simulink model "Week6"  (R2020b)
settings: Solver=VariableStepAuto  StartTime=0.0  StopTime=5  MaxStep=1e-4  RelTol=1e-3
undefined symbols (not defined in the file or in its folder): Capacitor, Run, Start
libraries: powerlib x9
settings Model: Creator=emman  LastModifiedBy=emman

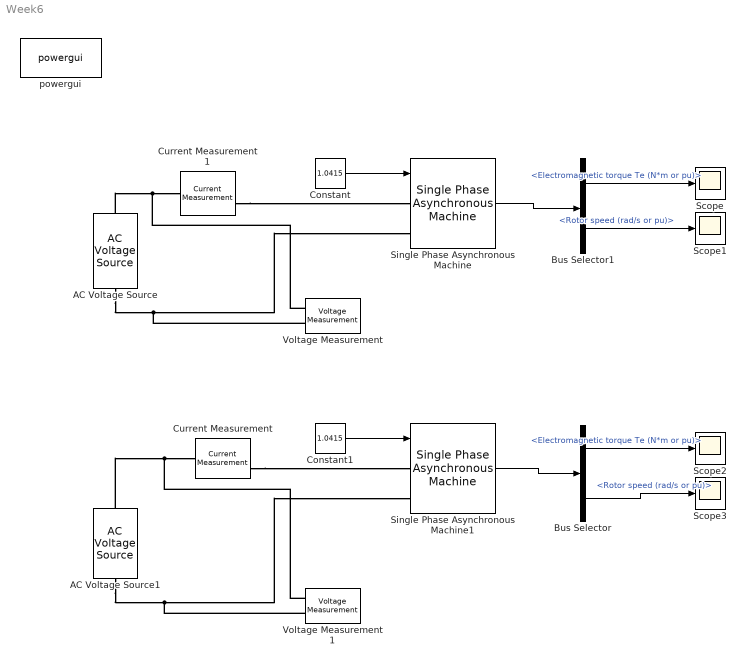
== system Week6 ==
  AC Voltage Source : powerlib/Electrical Sources/AC Voltage Source  Amplitude=110*sqrt(2)  Phase=90  Frequency=60  SampleTime=0  Measurements=None  BusType=swing  Pref=10e3  Qref=0  Qmin=-inf  Qmax=+inf
  AC Voltage Source1 : powerlib/Electrical Sources/AC Voltage Source  Amplitude=110*sqrt(2)  Phase=90  Frequency=60  SampleTime=0  Measurements=None  BusType=swing  Pref=10e3  Qref=0  Qmin=-inf  Qmax=+inf
  Bus Selector : BusSelector  OutputSignals=Mechanical.Electromagnetic torque Te (N*m or pu),Mechanical.Rotor speed (rad/s or pu)
  Bus Selector1 : BusSelector  OutputSignals=Mechanical.Electromagnetic torque Te (N*m or pu),Mechanical.Rotor speed (rad/s or pu)
  Constant : Constant  Value=1.0415
  Constant1 : Constant  Value=1.0415
  Current Measurement : powerlib/Measurements/Current Measurement  PhasorSimulation=off  OutputType=Complex  PSBequivalent=0
  Current Measurement1 : powerlib/Measurements/Current Measurement  PhasorSimulation=off  OutputType=Complex  PSBequivalent=0
  Scope{,1..3} (4 alike) : Scope
  Single Phase Asynchronous Machine : powerlib/Machines/Single Phase Asynchronous Machine  MechanicalLoad=Torque Tm  UNITS=SI  MachineType=Capacitor-Start  MeasurementBus=off  NominalParameters="[0.25*746  110  60]"  MainWindingStator="[2.02  7.4e-3]"  MainWindingRotor="[4.12  5.6e-3]"  MutualInductance=0.177  AuxiliaryWinding="[7.14  8.54e-3]"  Mechanical="[0.0146  0  2 1.18]"  CapacitorStart="[2.15  255e-6]"  CapacitorRun="[18  21.1e-6]"  DisconnectionSpeed=75  InitialSpeed=0  DataType=SI  TsPowergui=0  TsBlock=-1
      settings: SourceProductBaseCode=PS
  Single Phase Asynchronous Machine1 : powerlib/Machines/Single Phase Asynchronous Machine  MechanicalLoad=Torque Tm  UNITS=SI  MachineType=Capacitor-Start-Run  MeasurementBus=off  NominalParameters="[ .25*746  110  60]"  MainWindingStator="[2.02  7.4e-3]"  MainWindingRotor="[4.12  5.6e-3]"  MutualInductance=0.177  AuxiliaryWinding="[7.14  8.54e-3]"  Mechanical="[0.0146  0  2 1.18]"  CapacitorStart="[2.15  255e-6]"  CapacitorRun="[18  21.1e-6]"  DisconnectionSpeed=75  InitialSpeed=0  DataType=SI  TsPowergui=0  TsBlock=-1
      settings: SourceProductBaseCode=PS
  Voltage Measurement : powerlib/Measurements/Voltage Measurement  PhasorSimulation=off  OutputType=Complex  PSBequivalent=0
  Voltage Measurement1 : powerlib/Measurements/Voltage Measurement  PhasorSimulation=off  OutputType=Complex  PSBequivalent=0
  powergui : powerlib/powergui  Priority=1  SimulationMode=Continuous  SampleTime=50e-6  frequency=60  Iterations=50  frequencyindice=60  Pbase=100e6  ErrMax=1e-4  UnitsV=kV  UnitsW=MW  buscounter=0  FunctionMessages=off  echomessages=off  EnableUseOfTLC=off  CurrentSourceSwitches=off  DisableSnubberDevices=off  DisableRonSwitches=off  DisableVfSwitches=off  DisplayEquations=off  AutomaticDiscreteSolvers=off  SolverType=Tustin/Backward Euler (TBE)  Interpol=off  ExternalGateDelay=off  methode=off  Ts=100  x0status=blocks  SPID=on  SwTol=0  HookPort=off  NonlinearTolerance=1e-4  nMaxIteration=100  ContinueOnMaxIteration=off  RestoreLinks=warning  ResistiveCurrentMeasurement=off  Frange=[0:2:500]  Ylog=off  Xlog=on  ShowGrid=off  save=off  variable=ZData  structure=0  ZoomFFT=off  StartTime=0.0  cycles=1  DisplayStyle=1  fundamental=60  FreqAxis=off  MaxFrequency=1000  frequencyindicesteady=1  RmsSteady=1  display=off
  wires:
  Single Phase Asynchronous Machine/1 -> Bus Selector1/1
  Single Phase Asynchronous Machine1/1 -> Bus Selector/1
  Bus Selector/2 -> Scope3/1  "<Rotor speed (rad/s or pu)>"
  Bus Selector1/1 -> Scope/1  "<Electromagnetic torque Te (N*m or pu)>"
  Constant/1 -> Single Phase Asynchronous Machine/1
  Constant1/1 -> Single Phase Asynchronous Machine1/1
  Bus Selector/1 -> Scope2/1  "<Electromagnetic torque Te (N*m or pu)>"
  Bus Selector1/2 -> Scope1/1  "<Rotor speed (rad/s or pu)>"
  connections:
  AC Voltage Source/LConn1 -- Voltage Measurement/LConn2 -- Single Phase Asynchronous Machine/LConn2
  AC Voltage Source1/LConn1 -- Voltage Measurement1/LConn2 -- Single Phase Asynchronous Machine1/LConn2
  AC Voltage Source1/RConn1 -- Voltage Measurement1/LConn1 -- Current Measurement/LConn1
  Current Measurement/RConn1 -- Single Phase Asynchronous Machine1/LConn1
  AC Voltage Source/RConn1 -- Voltage Measurement/LConn1 -- Current Measurement1/LConn1
  Current Measurement1/RConn1 -- Single Phase Asynchronous Machine/LConn1
